simulink model "week1_problem5"  (R2020b)
settings: Solver=VariableStepAuto  StartTime=0.0  StopTime=10.0  RelTol=1e-3
model workspace (MAT data in the model file):
  C = Simulink.Parameter
  C.Value = 1e-06
  C.DataType = 'auto'
  C.Dimensions = [1 1]
  R = Simulink.Parameter
  R.Value = 10
  R.DataType = 'auto'
  R.Dimensions = [1 1]
settings Model: Creator=gokul  LastModifiedBy=gokul

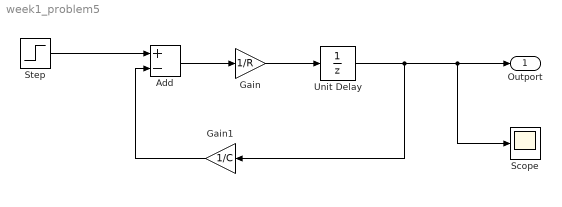
== system week1_problem5 ==
  Add : Sum  Inputs=+-
  Gain : Gain  Gain=1/R
  Gain1 : Gain  Gain=1/C
  Scope : Scope
  Step : Step  After=12  SampleTime=0
  Unit Delay : UnitDelay  SampleTime=-1  HasFrameUpgradeWarning=on
  Outport : Outport
  wires:
  Step/1 -> Add/1
  Add/1 -> Gain/1
  Gain/1 -> Unit Delay/1
  Unit Delay/1 -> Gain1/1, Scope/1, Outport/1
  Gain1/1 -> Add/2
